simulink model "ABS_Control_Logic_Unit"  (R2025a)
settings: Solver=VariableStepAuto  StartTime=0.0  StopTime=20  RelTol=1e-3
libraries: SignalEditorBlockLib x1
settings Model: Creator=Rudransh  LastModifiedBy=Rudransh

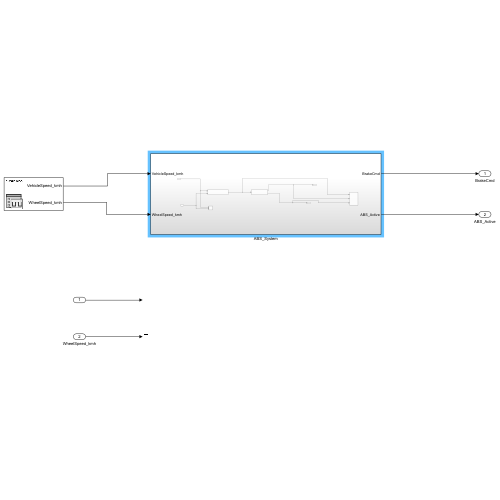
[thumbnail: Simulink's stored preview of the top-level diagram]
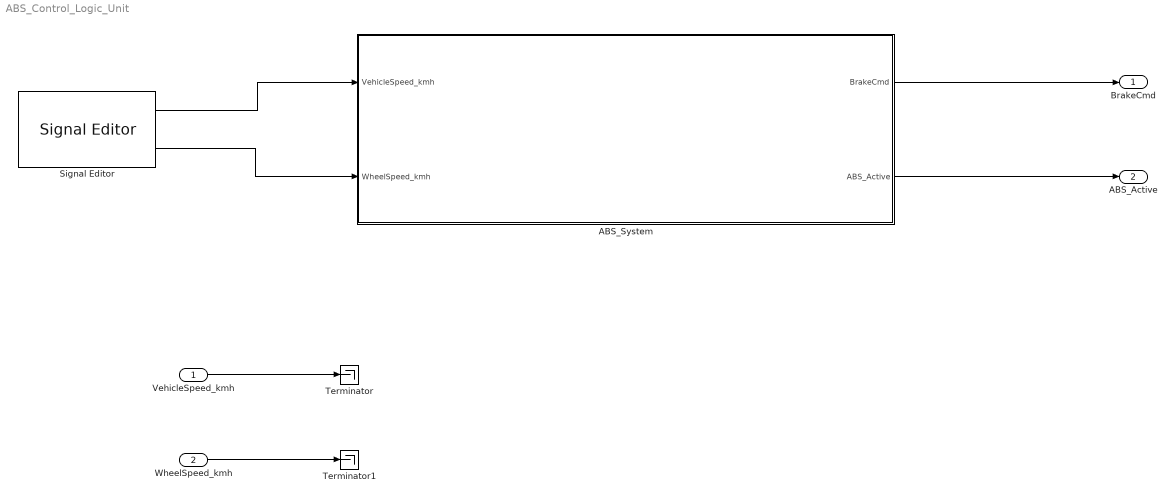
== system ABS_Control_Logic_Unit ==
  VehicleSpeed_kmh : Inport  OutDataTypeStr=double
  WheelSpeed_kmh : Inport  Port=2  OutDataTypeStr=double
  ABS_System : Subsystem
  Signal Editor : SignalEditorBlockLib/Signal Editor  FileName=C:\Projects_ESD\AUTOSAR_CARSYSTEM\ABS_Control_Logic\Scenario\Scenario1.mat  ActiveScenario=Scenario  ActiveSignal=VehicleSpeed_kmh  IsBus=off  OutputBusObjectStr=Bus: BusObject  SampleTime=0  ZeroCross=off  OutputAfterFinalValue=Setting to zero  Unit=inherit  PreserveSignalName=on  ApplySigPropsToAllScenarios=on  ApplySigPropsToAllSignals=off  SignalPropertySource=Dialog parameters
  Terminator : Terminator
  Terminator1 : Terminator
  BrakeCmd : Outport
  ABS_Active : Outport  Port=2  OutDataTypeStr=boolean
  wires:
  ABS_System/1(BrakeCmd) -> BrakeCmd/1
  ABS_System/2(ABS_Active) -> ABS_Active/1
  Signal Editor/1 -> ABS_System/1(VehicleSpeed_kmh)
  Signal Editor/2 -> ABS_System/2(WheelSpeed_kmh)
  WheelSpeed_kmh/1 -> Terminator1/1
  VehicleSpeed_kmh/1 -> Terminator/1

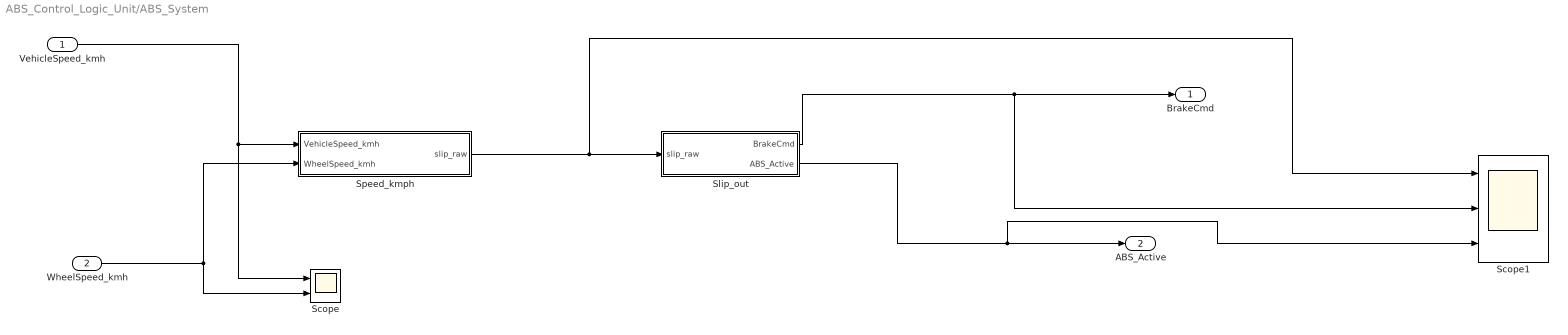
== system ABS_Control_Logic_Unit/ABS_System ==
  VehicleSpeed_kmh : Inport
  WheelSpeed_kmh : Inport  Port=2
  Scope : Scope  NumInputPorts=2
      settings: Title=VehicleSpeed  ActiveDisplayYMinimum=-9.9999999999999982  ActiveDisplayYMaximum=90
  Scope1 : Scope  NumInputPorts=3
      settings: ActiveDisplayString=3  Title=ABS_Active  ActiveDisplayYMinimum=0  ActiveDisplayYMaximum=1
  Slip_out : Subsystem
  Speed_kmph : Subsystem
  BrakeCmd : Outport
  ABS_Active : Outport  Port=2
  wires:
  Slip_out/2(ABS_Active) -> ABS_Active/1, Scope1/3
  Speed_kmph/1(slip_raw) -> Slip_out/1(slip_raw), Scope1/1
  Slip_out/1(BrakeCmd) -> BrakeCmd/1, Scope1/2
  WheelSpeed_kmh/1 -> Scope/2, Speed_kmph/2(WheelSpeed_kmh)
  VehicleSpeed_kmh/1 -> Scope/1, Speed_kmph/1(VehicleSpeed_kmh)

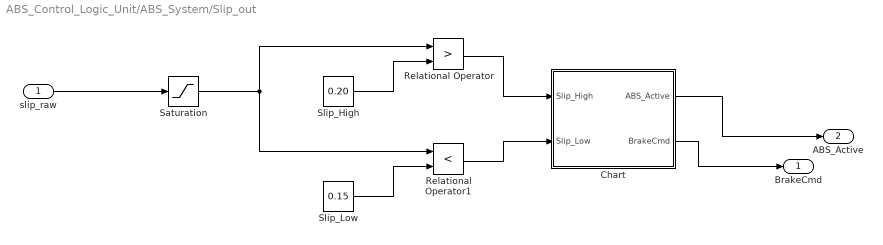
== system ABS_Control_Logic_Unit/ABS_System/Slip_out ==
  slip_raw : Inport
  Chart : Stateflow chart  TreatAsAtomicUnit=on
  Relational Operator : RelationalOperator  Operator=>  OutDataTypeStr=boolean  RndMeth=Simplest  InputSameDT=off
  Relational Operator1 : RelationalOperator  Operator=<  OutDataTypeStr=boolean  RndMeth=Simplest  InputSameDT=off
  Saturation : Saturate
  Slip_High : Constant  Value=0.20  VectorParams1D=off  OutDataTypeStr=double
  Slip_Low : Constant  Value=0.15
  BrakeCmd : Outport
  ABS_Active : Outport  Port=2
  wires:
  Relational Operator1/1 -> Chart/2(Slip_Low)
  Chart/1(ABS_Active) -> ABS_Active/1
  Saturation/1 -> Relational Operator1/1, Relational Operator/1
  Relational Operator/1 -> Chart/1(Slip_High)
  Slip_High/1 -> Relational Operator/2
  Slip_Low/1 -> Relational Operator1/2
  slip_raw/1 -> Saturation/1
  Chart/2(BrakeCmd) -> BrakeCmd/1

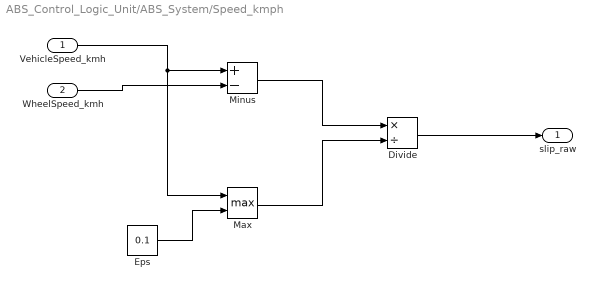
== system ABS_Control_Logic_Unit/ABS_System/Speed_kmph ==
  VehicleSpeed_kmh : Inport
  WheelSpeed_kmh : Inport  Port=2
  Divide : Product  Inputs=*/
  Eps : Constant  Value=0.1
  Max : MinMax  Function=max  Inputs=2
  Minus : Sum  Inputs=+-
  slip_raw : Outport
  wires:
  Minus/1 -> Divide/1
  Divide/1 -> slip_raw/1
  VehicleSpeed_kmh/1 -> Max/1, Minus/1
  Max/1 -> Divide/2
  Eps/1 -> Max/2
  WheelSpeed_kmh/1 -> Minus/2

== stateflow chart ABS_Control_Logic_Unit/ABS_System/Slip_out/Chart ==
  state Idle_State
    BrakeCmd = 1.0;
    ABS_Active = false;
  state Apply_State
    BrakeCmd = 1.0;
    ABS_Active = true;
  state Release_State
    BrakeCmd = 0.3;
    ABS_Active = true;
  (default) -> Idle_State
  Release_State -> Idle_State [order 2] : [after(0.1,sec) && Slip_Low]
  Idle_State -> Apply_State : [Slip_High]
  Apply_State -> Release_State : after(0.1,sec) %Release
  Release_State -> Apply_State [order 1] : [after(0.1,sec) && Slip_High]
  data: Slip_High input; Slip_Low input; ABS_Active output; BrakeCmd output
